simulink model "sim_model"  (R2015b)
settings: Solver=FixedStepDiscrete  SolverMode=SingleTasking  StartTime=0.0  StopTime=sim_len  FixedStep=1  RelTol=1e-3
undefined symbols (not defined in the file): A, B, C, ir_matrix, modulator_reg_1_address, modulator_reg_1_default, modulator_reg_1_num_bits, N_sub
libraries: xbsIndex_r4 x3875
(part 192 of 193)

== system sim_model/channelizer/poly_phase_filter1/filter_pipeline_89_taps3/8_taps6/one_tab_1/ring_buffer_1 ==
  reset_in : Inport
  enable_in : Inport  Port=2
  data_in : Inport  Port=3
  Register : xbsIndex_r4/Register  init=init(1)  rst=on  en=on  dbl_ovrd=off  block_type=register
  Register1 : xbsIndex_r4/Register  init=init(2)  rst=on  en=on  dbl_ovrd=off  block_type=register
  Register2 : xbsIndex_r4/Register  init=init(3)  rst=on  en=on  dbl_ovrd=off  block_type=register
  Register3 : xbsIndex_r4/Register  init=init(4)  rst=on  en=on  dbl_ovrd=off  block_type=register
  Register4 : xbsIndex_r4/Register  init=init(5)  rst=on  en=on  dbl_ovrd=off  block_type=register
  Register5 : xbsIndex_r4/Register  init=init(6)  rst=on  en=on  dbl_ovrd=off  block_type=register
  Register6 : xbsIndex_r4/Register  init=init(7)  rst=on  en=on  dbl_ovrd=off  block_type=register
  Register7 : xbsIndex_r4/Register  init=init(8)  rst=on  en=on  dbl_ovrd=off  block_type=register
  data_out : Outport
  wires:
  Register/1 -> Register1/1
  enable_in/1 -> Register7/3, Register6/3, Register5/3, Register4/3, Register3/3, Register2/3, Register1/3, Register/3
  Register7/1 -> data_out/1
  Register1/1 -> Register2/1
  Register2/1 -> Register3/1
  Register3/1 -> Register4/1
  Register5/1 -> Register6/1
  Register6/1 -> Register7/1
  Register4/1 -> Register5/1
  reset_in/1 -> Register/2, Register1/2, Register2/2, Register3/2, Register4/2, Register7/2, Register6/2, Register5/2
  data_in/1 -> Register/1

== system sim_model/channelizer/poly_phase_filter1/filter_pipeline_89_taps3/8_taps6/one_tab_1/ring_buffer_8 ==
  reset_in : Inport
  enable_in : Inport  Port=2
  data_in : Inport  Port=3
  Register : xbsIndex_r4/Register  init=init(1)  rst=on  en=on  dbl_ovrd=off  block_type=register
  Register1 : xbsIndex_r4/Register  init=init(2)  rst=on  en=on  dbl_ovrd=off  block_type=register
  Register2 : xbsIndex_r4/Register  init=init(3)  rst=on  en=on  dbl_ovrd=off  block_type=register
  Register3 : xbsIndex_r4/Register  init=init(4)  rst=on  en=on  dbl_ovrd=off  block_type=register
  Register4 : xbsIndex_r4/Register  init=init(5)  rst=on  en=on  dbl_ovrd=off  block_type=register
  Register5 : xbsIndex_r4/Register  init=init(6)  rst=on  en=on  dbl_ovrd=off  block_type=register
  Register6 : xbsIndex_r4/Register  init=init(7)  rst=on  en=on  dbl_ovrd=off  block_type=register
  Register7 : xbsIndex_r4/Register  init=init(8)  rst=on  en=on  dbl_ovrd=off  block_type=register
  data_out : Outport
  wires:
  Register/1 -> Register1/1
  enable_in/1 -> Register7/3, Register6/3, Register5/3, Register4/3, Register3/3, Register2/3, Register1/3, Register/3
  Register7/1 -> data_out/1
  Register1/1 -> Register2/1
  Register2/1 -> Register3/1
  Register3/1 -> Register4/1
  Register5/1 -> Register6/1
  Register6/1 -> Register7/1
  Register4/1 -> Register5/1
  reset_in/1 -> Register/2, Register1/2, Register2/2, Register3/2, Register4/2, Register7/2, Register6/2, Register5/2
  data_in/1 -> Register/1

== system sim_model/channelizer/poly_phase_filter1/filter_pipeline_89_taps3/8_taps6/one_tab_2/ring_buffer_1 ==
  reset_in : Inport
  enable_in : Inport  Port=2
  data_in : Inport  Port=3
  Register : xbsIndex_r4/Register  init=init(1)  rst=on  en=on  dbl_ovrd=off  block_type=register
  Register1 : xbsIndex_r4/Register  init=init(2)  rst=on  en=on  dbl_ovrd=off  block_type=register
  Register2 : xbsIndex_r4/Register  init=init(3)  rst=on  en=on  dbl_ovrd=off  block_type=register
  Register3 : xbsIndex_r4/Register  init=init(4)  rst=on  en=on  dbl_ovrd=off  block_type=register
  Register4 : xbsIndex_r4/Register  init=init(5)  rst=on  en=on  dbl_ovrd=off  block_type=register
  Register5 : xbsIndex_r4/Register  init=init(6)  rst=on  en=on  dbl_ovrd=off  block_type=register
  Register6 : xbsIndex_r4/Register  init=init(7)  rst=on  en=on  dbl_ovrd=off  block_type=register
  Register7 : xbsIndex_r4/Register  init=init(8)  rst=on  en=on  dbl_ovrd=off  block_type=register
  data_out : Outport
  wires:
  Register/1 -> Register1/1
  enable_in/1 -> Register7/3, Register6/3, Register5/3, Register4/3, Register3/3, Register2/3, Register1/3, Register/3
  Register7/1 -> data_out/1
  Register1/1 -> Register2/1
  Register2/1 -> Register3/1
  Register3/1 -> Register4/1
  Register5/1 -> Register6/1
  Register6/1 -> Register7/1
  Register4/1 -> Register5/1
  reset_in/1 -> Register/2, Register1/2, Register2/2, Register3/2, Register4/2, Register7/2, Register6/2, Register5/2
  data_in/1 -> Register/1

== system sim_model/channelizer/poly_phase_filter1/filter_pipeline_89_taps3/8_taps6/one_tab_2/ring_buffer_8 ==
  reset_in : Inport
  enable_in : Inport  Port=2
  data_in : Inport  Port=3
  Register : xbsIndex_r4/Register  init=init(1)  rst=on  en=on  dbl_ovrd=off  block_type=register
  Register1 : xbsIndex_r4/Register  init=init(2)  rst=on  en=on  dbl_ovrd=off  block_type=register
  Register2 : xbsIndex_r4/Register  init=init(3)  rst=on  en=on  dbl_ovrd=off  block_type=register
  Register3 : xbsIndex_r4/Register  init=init(4)  rst=on  en=on  dbl_ovrd=off  block_type=register
  Register4 : xbsIndex_r4/Register  init=init(5)  rst=on  en=on  dbl_ovrd=off  block_type=register
  Register5 : xbsIndex_r4/Register  init=init(6)  rst=on  en=on  dbl_ovrd=off  block_type=register
  Register6 : xbsIndex_r4/Register  init=init(7)  rst=on  en=on  dbl_ovrd=off  block_type=register
  Register7 : xbsIndex_r4/Register  init=init(8)  rst=on  en=on  dbl_ovrd=off  block_type=register
  data_out : Outport
  wires:
  Register/1 -> Register1/1
  enable_in/1 -> Register7/3, Register6/3, Register5/3, Register4/3, Register3/3, Register2/3, Register1/3, Register/3
  Register7/1 -> data_out/1
  Register1/1 -> Register2/1
  Register2/1 -> Register3/1
  Register3/1 -> Register4/1
  Register5/1 -> Register6/1
  Register6/1 -> Register7/1
  Register4/1 -> Register5/1
  reset_in/1 -> Register/2, Register1/2, Register2/2, Register3/2, Register4/2, Register7/2, Register6/2, Register5/2
  data_in/1 -> Register/1

== system sim_model/channelizer/poly_phase_filter1/filter_pipeline_89_taps3/8_taps6/one_tab_3/ring_buffer_1 ==
  reset_in : Inport
  enable_in : Inport  Port=2
  data_in : Inport  Port=3
  Register : xbsIndex_r4/Register  init=init(1)  rst=on  en=on  dbl_ovrd=off  block_type=register
  Register1 : xbsIndex_r4/Register  init=init(2)  rst=on  en=on  dbl_ovrd=off  block_type=register
  Register2 : xbsIndex_r4/Register  init=init(3)  rst=on  en=on  dbl_ovrd=off  block_type=register
  Register3 : xbsIndex_r4/Register  init=init(4)  rst=on  en=on  dbl_ovrd=off  block_type=register
  Register4 : xbsIndex_r4/Register  init=init(5)  rst=on  en=on  dbl_ovrd=off  block_type=register
  Register5 : xbsIndex_r4/Register  init=init(6)  rst=on  en=on  dbl_ovrd=off  block_type=register
  Register6 : xbsIndex_r4/Register  init=init(7)  rst=on  en=on  dbl_ovrd=off  block_type=register
  Register7 : xbsIndex_r4/Register  init=init(8)  rst=on  en=on  dbl_ovrd=off  block_type=register
  data_out : Outport
  wires:
  Register/1 -> Register1/1
  enable_in/1 -> Register7/3, Register6/3, Register5/3, Register4/3, Register3/3, Register2/3, Register1/3, Register/3
  Register7/1 -> data_out/1
  Register1/1 -> Register2/1
  Register2/1 -> Register3/1
  Register3/1 -> Register4/1
  Register5/1 -> Register6/1
  Register6/1 -> Register7/1
  Register4/1 -> Register5/1
  reset_in/1 -> Register/2, Register1/2, Register2/2, Register3/2, Register4/2, Register7/2, Register6/2, Register5/2
  data_in/1 -> Register/1

== system sim_model/channelizer/poly_phase_filter1/filter_pipeline_89_taps3/8_taps6/one_tab_3/ring_buffer_8 ==
  reset_in : Inport
  enable_in : Inport  Port=2
  data_in : Inport  Port=3
  Register : xbsIndex_r4/Register  init=init(1)  rst=on  en=on  dbl_ovrd=off  block_type=register
  Register1 : xbsIndex_r4/Register  init=init(2)  rst=on  en=on  dbl_ovrd=off  block_type=register
  Register2 : xbsIndex_r4/Register  init=init(3)  rst=on  en=on  dbl_ovrd=off  block_type=register
  Register3 : xbsIndex_r4/Register  init=init(4)  rst=on  en=on  dbl_ovrd=off  block_type=register
  Register4 : xbsIndex_r4/Register  init=init(5)  rst=on  en=on  dbl_ovrd=off  block_type=register
  Register5 : xbsIndex_r4/Register  init=init(6)  rst=on  en=on  dbl_ovrd=off  block_type=register
  Register6 : xbsIndex_r4/Register  init=init(7)  rst=on  en=on  dbl_ovrd=off  block_type=register
  Register7 : xbsIndex_r4/Register  init=init(8)  rst=on  en=on  dbl_ovrd=off  block_type=register
  data_out : Outport
  wires:
  Register/1 -> Register1/1
  enable_in/1 -> Register7/3, Register6/3, Register5/3, Register4/3, Register3/3, Register2/3, Register1/3, Register/3
  Register7/1 -> data_out/1
  Register1/1 -> Register2/1
  Register2/1 -> Register3/1
  Register3/1 -> Register4/1
  Register5/1 -> Register6/1
  Register6/1 -> Register7/1
  Register4/1 -> Register5/1
  reset_in/1 -> Register/2, Register1/2, Register2/2, Register3/2, Register4/2, Register7/2, Register6/2, Register5/2
  data_in/1 -> Register/1

== system sim_model/channelizer/poly_phase_filter1/filter_pipeline_89_taps3/8_taps6/one_tab_4/ring_buffer_1 ==
  reset_in : Inport
  enable_in : Inport  Port=2
  data_in : Inport  Port=3
  Register : xbsIndex_r4/Register  init=init(1)  rst=on  en=on  dbl_ovrd=off  block_type=register
  Register1 : xbsIndex_r4/Register  init=init(2)  rst=on  en=on  dbl_ovrd=off  block_type=register
  Register2 : xbsIndex_r4/Register  init=init(3)  rst=on  en=on  dbl_ovrd=off  block_type=register
  Register3 : xbsIndex_r4/Register  init=init(4)  rst=on  en=on  dbl_ovrd=off  block_type=register
  Register4 : xbsIndex_r4/Register  init=init(5)  rst=on  en=on  dbl_ovrd=off  block_type=register
  Register5 : xbsIndex_r4/Register  init=init(6)  rst=on  en=on  dbl_ovrd=off  block_type=register
  Register6 : xbsIndex_r4/Register  init=init(7)  rst=on  en=on  dbl_ovrd=off  block_type=register
  Register7 : xbsIndex_r4/Register  init=init(8)  rst=on  en=on  dbl_ovrd=off  block_type=register
  data_out : Outport
  wires:
  Register/1 -> Register1/1
  enable_in/1 -> Register7/3, Register6/3, Register5/3, Register4/3, Register3/3, Register2/3, Register1/3, Register/3
  Register7/1 -> data_out/1
  Register1/1 -> Register2/1
  Register2/1 -> Register3/1
  Register3/1 -> Register4/1
  Register5/1 -> Register6/1
  Register6/1 -> Register7/1
  Register4/1 -> Register5/1
  reset_in/1 -> Register/2, Register1/2, Register2/2, Register3/2, Register4/2, Register7/2, Register6/2, Register5/2
  data_in/1 -> Register/1

== system sim_model/channelizer/poly_phase_filter1/filter_pipeline_89_taps3/8_taps6/one_tab_4/ring_buffer_8 ==
  reset_in : Inport
  enable_in : Inport  Port=2
  data_in : Inport  Port=3
  Register : xbsIndex_r4/Register  init=init(1)  rst=on  en=on  dbl_ovrd=off  block_type=register
  Register1 : xbsIndex_r4/Register  init=init(2)  rst=on  en=on  dbl_ovrd=off  block_type=register
  Register2 : xbsIndex_r4/Register  init=init(3)  rst=on  en=on  dbl_ovrd=off  block_type=register
  Register3 : xbsIndex_r4/Register  init=init(4)  rst=on  en=on  dbl_ovrd=off  block_type=register
  Register4 : xbsIndex_r4/Register  init=init(5)  rst=on  en=on  dbl_ovrd=off  block_type=register
  Register5 : xbsIndex_r4/Register  init=init(6)  rst=on  en=on  dbl_ovrd=off  block_type=register
  Register6 : xbsIndex_r4/Register  init=init(7)  rst=on  en=on  dbl_ovrd=off  block_type=register
  Register7 : xbsIndex_r4/Register  init=init(8)  rst=on  en=on  dbl_ovrd=off  block_type=register
  data_out : Outport
  wires:
  Register/1 -> Register1/1
  enable_in/1 -> Register7/3, Register6/3, Register5/3, Register4/3, Register3/3, Register2/3, Register1/3, Register/3
  Register7/1 -> data_out/1
  Register1/1 -> Register2/1
  Register2/1 -> Register3/1
  Register3/1 -> Register4/1
  Register5/1 -> Register6/1
  Register6/1 -> Register7/1
  Register4/1 -> Register5/1
  reset_in/1 -> Register/2, Register1/2, Register2/2, Register3/2, Register4/2, Register7/2, Register6/2, Register5/2
  data_in/1 -> Register/1

== system sim_model/channelizer/poly_phase_filter1/filter_pipeline_89_taps3/8_taps6/one_tab_5/ring_buffer_1 ==
  reset_in : Inport
  enable_in : Inport  Port=2
  data_in : Inport  Port=3
  Register : xbsIndex_r4/Register  init=init(1)  rst=on  en=on  dbl_ovrd=off  block_type=register
  Register1 : xbsIndex_r4/Register  init=init(2)  rst=on  en=on  dbl_ovrd=off  block_type=register
  Register2 : xbsIndex_r4/Register  init=init(3)  rst=on  en=on  dbl_ovrd=off  block_type=register
  Register3 : xbsIndex_r4/Register  init=init(4)  rst=on  en=on  dbl_ovrd=off  block_type=register
  Register4 : xbsIndex_r4/Register  init=init(5)  rst=on  en=on  dbl_ovrd=off  block_type=register
  Register5 : xbsIndex_r4/Register  init=init(6)  rst=on  en=on  dbl_ovrd=off  block_type=register
  Register6 : xbsIndex_r4/Register  init=init(7)  rst=on  en=on  dbl_ovrd=off  block_type=register
  Register7 : xbsIndex_r4/Register  init=init(8)  rst=on  en=on  dbl_ovrd=off  block_type=register
  data_out : Outport
  wires:
  Register/1 -> Register1/1
  enable_in/1 -> Register7/3, Register6/3, Register5/3, Register4/3, Register3/3, Register2/3, Register1/3, Register/3
  Register7/1 -> data_out/1
  Register1/1 -> Register2/1
  Register2/1 -> Register3/1
  Register3/1 -> Register4/1
  Register5/1 -> Register6/1
  Register6/1 -> Register7/1
  Register4/1 -> Register5/1
  reset_in/1 -> Register/2, Register1/2, Register2/2, Register3/2, Register4/2, Register7/2, Register6/2, Register5/2
  data_in/1 -> Register/1

== system sim_model/channelizer/poly_phase_filter1/filter_pipeline_89_taps3/8_taps6/one_tab_5/ring_buffer_8 ==
  reset_in : Inport
  enable_in : Inport  Port=2
  data_in : Inport  Port=3
  Register : xbsIndex_r4/Register  init=init(1)  rst=on  en=on  dbl_ovrd=off  block_type=register
  Register1 : xbsIndex_r4/Register  init=init(2)  rst=on  en=on  dbl_ovrd=off  block_type=register
  Register2 : xbsIndex_r4/Register  init=init(3)  rst=on  en=on  dbl_ovrd=off  block_type=register
  Register3 : xbsIndex_r4/Register  init=init(4)  rst=on  en=on  dbl_ovrd=off  block_type=register
  Register4 : xbsIndex_r4/Register  init=init(5)  rst=on  en=on  dbl_ovrd=off  block_type=register
  Register5 : xbsIndex_r4/Register  init=init(6)  rst=on  en=on  dbl_ovrd=off  block_type=register
  Register6 : xbsIndex_r4/Register  init=init(7)  rst=on  en=on  dbl_ovrd=off  block_type=register
  Register7 : xbsIndex_r4/Register  init=init(8)  rst=on  en=on  dbl_ovrd=off  block_type=register
  data_out : Outport
  wires:
  Register/1 -> Register1/1
  enable_in/1 -> Register7/3, Register6/3, Register5/3, Register4/3, Register3/3, Register2/3, Register1/3, Register/3
  Register7/1 -> data_out/1
  Register1/1 -> Register2/1
  Register2/1 -> Register3/1
  Register3/1 -> Register4/1
  Register5/1 -> Register6/1
  Register6/1 -> Register7/1
  Register4/1 -> Register5/1
  reset_in/1 -> Register/2, Register1/2, Register2/2, Register3/2, Register4/2, Register7/2, Register6/2, Register5/2
  data_in/1 -> Register/1

== system sim_model/channelizer/poly_phase_filter1/filter_pipeline_89_taps3/8_taps6/one_tab_6/ring_buffer_1 ==
  reset_in : Inport
  enable_in : Inport  Port=2
  data_in : Inport  Port=3
  Register : xbsIndex_r4/Register  init=init(1)  rst=on  en=on  dbl_ovrd=off  block_type=register
  Register1 : xbsIndex_r4/Register  init=init(2)  rst=on  en=on  dbl_ovrd=off  block_type=register
  Register2 : xbsIndex_r4/Register  init=init(3)  rst=on  en=on  dbl_ovrd=off  block_type=register
  Register3 : xbsIndex_r4/Register  init=init(4)  rst=on  en=on  dbl_ovrd=off  block_type=register
  Register4 : xbsIndex_r4/Register  init=init(5)  rst=on  en=on  dbl_ovrd=off  block_type=register
  Register5 : xbsIndex_r4/Register  init=init(6)  rst=on  en=on  dbl_ovrd=off  block_type=register
  Register6 : xbsIndex_r4/Register  init=init(7)  rst=on  en=on  dbl_ovrd=off  block_type=register
  Register7 : xbsIndex_r4/Register  init=init(8)  rst=on  en=on  dbl_ovrd=off  block_type=register
  data_out : Outport
  wires:
  Register/1 -> Register1/1
  enable_in/1 -> Register7/3, Register6/3, Register5/3, Register4/3, Register3/3, Register2/3, Register1/3, Register/3
  Register7/1 -> data_out/1
  Register1/1 -> Register2/1
  Register2/1 -> Register3/1
  Register3/1 -> Register4/1
  Register5/1 -> Register6/1
  Register6/1 -> Register7/1
  Register4/1 -> Register5/1
  reset_in/1 -> Register/2, Register1/2, Register2/2, Register3/2, Register4/2, Register7/2, Register6/2, Register5/2
  data_in/1 -> Register/1

== system sim_model/channelizer/poly_phase_filter1/filter_pipeline_89_taps3/8_taps6/one_tab_6/ring_buffer_8 ==
  reset_in : Inport
  enable_in : Inport  Port=2
  data_in : Inport  Port=3
  Register : xbsIndex_r4/Register  init=init(1)  rst=on  en=on  dbl_ovrd=off  block_type=register
  Register1 : xbsIndex_r4/Register  init=init(2)  rst=on  en=on  dbl_ovrd=off  block_type=register
  Register2 : xbsIndex_r4/Register  init=init(3)  rst=on  en=on  dbl_ovrd=off  block_type=register
  Register3 : xbsIndex_r4/Register  init=init(4)  rst=on  en=on  dbl_ovrd=off  block_type=register
  Register4 : xbsIndex_r4/Register  init=init(5)  rst=on  en=on  dbl_ovrd=off  block_type=register
  Register5 : xbsIndex_r4/Register  init=init(6)  rst=on  en=on  dbl_ovrd=off  block_type=register
  Register6 : xbsIndex_r4/Register  init=init(7)  rst=on  en=on  dbl_ovrd=off  block_type=register
  Register7 : xbsIndex_r4/Register  init=init(8)  rst=on  en=on  dbl_ovrd=off  block_type=register
  data_out : Outport
  wires:
  Register/1 -> Register1/1
  enable_in/1 -> Register7/3, Register6/3, Register5/3, Register4/3, Register3/3, Register2/3, Register1/3, Register/3
  Register7/1 -> data_out/1
  Register1/1 -> Register2/1
  Register2/1 -> Register3/1
  Register3/1 -> Register4/1
  Register5/1 -> Register6/1
  Register6/1 -> Register7/1
  Register4/1 -> Register5/1
  reset_in/1 -> Register/2, Register1/2, Register2/2, Register3/2, Register4/2, Register7/2, Register6/2, Register5/2
  data_in/1 -> Register/1

== system sim_model/channelizer/poly_phase_filter1/filter_pipeline_89_taps3/8_taps6/one_tab_7/ring_buffer_1 ==
  reset_in : Inport
  enable_in : Inport  Port=2
  data_in : Inport  Port=3
  Register : xbsIndex_r4/Register  init=init(1)  rst=on  en=on  dbl_ovrd=off  block_type=register
  Register1 : xbsIndex_r4/Register  init=init(2)  rst=on  en=on  dbl_ovrd=off  block_type=register
  Register2 : xbsIndex_r4/Register  init=init(3)  rst=on  en=on  dbl_ovrd=off  block_type=register
  Register3 : xbsIndex_r4/Register  init=init(4)  rst=on  en=on  dbl_ovrd=off  block_type=register
  Register4 : xbsIndex_r4/Register  init=init(5)  rst=on  en=on  dbl_ovrd=off  block_type=register
  Register5 : xbsIndex_r4/Register  init=init(6)  rst=on  en=on  dbl_ovrd=off  block_type=register
  Register6 : xbsIndex_r4/Register  init=init(7)  rst=on  en=on  dbl_ovrd=off  block_type=register
  Register7 : xbsIndex_r4/Register  init=init(8)  rst=on  en=on  dbl_ovrd=off  block_type=register
  data_out : Outport
  wires:
  Register/1 -> Register1/1
  enable_in/1 -> Register7/3, Register6/3, Register5/3, Register4/3, Register3/3, Register2/3, Register1/3, Register/3
  Register7/1 -> data_out/1
  Register1/1 -> Register2/1
  Register2/1 -> Register3/1
  Register3/1 -> Register4/1
  Register5/1 -> Register6/1
  Register6/1 -> Register7/1
  Register4/1 -> Register5/1
  reset_in/1 -> Register/2, Register1/2, Register2/2, Register3/2, Register4/2, Register7/2, Register6/2, Register5/2
  data_in/1 -> Register/1

== system sim_model/channelizer/poly_phase_filter1/filter_pipeline_89_taps3/8_taps6/one_tab_7/ring_buffer_8 ==
  reset_in : Inport
  enable_in : Inport  Port=2
  data_in : Inport  Port=3
  Register : xbsIndex_r4/Register  init=init(1)  rst=on  en=on  dbl_ovrd=off  block_type=register
  Register1 : xbsIndex_r4/Register  init=init(2)  rst=on  en=on  dbl_ovrd=off  block_type=register
  Register2 : xbsIndex_r4/Register  init=init(3)  rst=on  en=on  dbl_ovrd=off  block_type=register
  Register3 : xbsIndex_r4/Register  init=init(4)  rst=on  en=on  dbl_ovrd=off  block_type=register
  Register4 : xbsIndex_r4/Register  init=init(5)  rst=on  en=on  dbl_ovrd=off  block_type=register
  Register5 : xbsIndex_r4/Register  init=init(6)  rst=on  en=on  dbl_ovrd=off  block_type=register
  Register6 : xbsIndex_r4/Register  init=init(7)  rst=on  en=on  dbl_ovrd=off  block_type=register
  Register7 : xbsIndex_r4/Register  init=init(8)  rst=on  en=on  dbl_ovrd=off  block_type=register
  data_out : Outport
  wires:
  Register/1 -> Register1/1
  enable_in/1 -> Register7/3, Register6/3, Register5/3, Register4/3, Register3/3, Register2/3, Register1/3, Register/3
  Register7/1 -> data_out/1
  Register1/1 -> Register2/1
  Register2/1 -> Register3/1
  Register3/1 -> Register4/1
  Register5/1 -> Register6/1
  Register6/1 -> Register7/1
  Register4/1 -> Register5/1
  reset_in/1 -> Register/2, Register1/2, Register2/2, Register3/2, Register4/2, Register7/2, Register6/2, Register5/2
  data_in/1 -> Register/1

== system sim_model/channelizer/poly_phase_filter1/filter_pipeline_89_taps3/8_taps6/one_tab_8/ring_buffer_1 ==
  reset_in : Inport
  enable_in : Inport  Port=2
  data_in : Inport  Port=3
  Register : xbsIndex_r4/Register  init=init(1)  rst=on  en=on  dbl_ovrd=off  block_type=register
  Register1 : xbsIndex_r4/Register  init=init(2)  rst=on  en=on  dbl_ovrd=off  block_type=register
  Register2 : xbsIndex_r4/Register  init=init(3)  rst=on  en=on  dbl_ovrd=off  block_type=register
  Register3 : xbsIndex_r4/Register  init=init(4)  rst=on  en=on  dbl_ovrd=off  block_type=register
  Register4 : xbsIndex_r4/Register  init=init(5)  rst=on  en=on  dbl_ovrd=off  block_type=register
  Register5 : xbsIndex_r4/Register  init=init(6)  rst=on  en=on  dbl_ovrd=off  block_type=register
  Register6 : xbsIndex_r4/Register  init=init(7)  rst=on  en=on  dbl_ovrd=off  block_type=register
  Register7 : xbsIndex_r4/Register  init=init(8)  rst=on  en=on  dbl_ovrd=off  block_type=register
  data_out : Outport
  wires:
  Register/1 -> Register1/1
  enable_in/1 -> Register7/3, Register6/3, Register5/3, Register4/3, Register3/3, Register2/3, Register1/3, Register/3
  Register7/1 -> data_out/1
  Register1/1 -> Register2/1
  Register2/1 -> Register3/1
  Register3/1 -> Register4/1
  Register5/1 -> Register6/1
  Register6/1 -> Register7/1
  Register4/1 -> Register5/1
  reset_in/1 -> Register/2, Register1/2, Register2/2, Register3/2, Register4/2, Register7/2, Register6/2, Register5/2
  data_in/1 -> Register/1

== system sim_model/channelizer/poly_phase_filter1/filter_pipeline_89_taps3/8_taps6/one_tab_8/ring_buffer_8 ==
  reset_in : Inport
  enable_in : Inport  Port=2
  data_in : Inport  Port=3
  Register : xbsIndex_r4/Register  init=init(1)  rst=on  en=on  dbl_ovrd=off  block_type=register
  Register1 : xbsIndex_r4/Register  init=init(2)  rst=on  en=on  dbl_ovrd=off  block_type=register
  Register2 : xbsIndex_r4/Register  init=init(3)  rst=on  en=on  dbl_ovrd=off  block_type=register
  Register3 : xbsIndex_r4/Register  init=init(4)  rst=on  en=on  dbl_ovrd=off  block_type=register
  Register4 : xbsIndex_r4/Register  init=init(5)  rst=on  en=on  dbl_ovrd=off  block_type=register
  Register5 : xbsIndex_r4/Register  init=init(6)  rst=on  en=on  dbl_ovrd=off  block_type=register
  Register6 : xbsIndex_r4/Register  init=init(7)  rst=on  en=on  dbl_ovrd=off  block_type=register
  Register7 : xbsIndex_r4/Register  init=init(8)  rst=on  en=on  dbl_ovrd=off  block_type=register
  data_out : Outport
  wires:
  Register/1 -> Register1/1
  enable_in/1 -> Register7/3, Register6/3, Register5/3, Register4/3, Register3/3, Register2/3, Register1/3, Register/3
  Register7/1 -> data_out/1
  Register1/1 -> Register2/1
  Register2/1 -> Register3/1
  Register3/1 -> Register4/1
  Register5/1 -> Register6/1
  Register6/1 -> Register7/1
  Register4/1 -> Register5/1
  reset_in/1 -> Register/2, Register1/2, Register2/2, Register3/2, Register4/2, Register7/2, Register6/2, Register5/2
  data_in/1 -> Register/1

== system sim_model/channelizer/poly_phase_filter1/filter_pipeline_89_taps3/8_taps7/one_tab_1/ring_buffer_1 ==
  reset_in : Inport
  enable_in : Inport  Port=2
  data_in : Inport  Port=3
  Register : xbsIndex_r4/Register  init=init(1)  rst=on  en=on  dbl_ovrd=off  block_type=register
  Register1 : xbsIndex_r4/Register  init=init(2)  rst=on  en=on  dbl_ovrd=off  block_type=register
  Register2 : xbsIndex_r4/Register  init=init(3)  rst=on  en=on  dbl_ovrd=off  block_type=register
  Register3 : xbsIndex_r4/Register  init=init(4)  rst=on  en=on  dbl_ovrd=off  block_type=register
  Register4 : xbsIndex_r4/Register  init=init(5)  rst=on  en=on  dbl_ovrd=off  block_type=register
  Register5 : xbsIndex_r4/Register  init=init(6)  rst=on  en=on  dbl_ovrd=off  block_type=register
  Register6 : xbsIndex_r4/Register  init=init(7)  rst=on  en=on  dbl_ovrd=off  block_type=register
  Register7 : xbsIndex_r4/Register  init=init(8)  rst=on  en=on  dbl_ovrd=off  block_type=register
  data_out : Outport
  wires:
  Register/1 -> Register1/1
  enable_in/1 -> Register7/3, Register6/3, Register5/3, Register4/3, Register3/3, Register2/3, Register1/3, Register/3
  Register7/1 -> data_out/1
  Register1/1 -> Register2/1
  Register2/1 -> Register3/1
  Register3/1 -> Register4/1
  Register5/1 -> Register6/1
  Register6/1 -> Register7/1
  Register4/1 -> Register5/1
  reset_in/1 -> Register/2, Register1/2, Register2/2, Register3/2, Register4/2, Register7/2, Register6/2, Register5/2
  data_in/1 -> Register/1

== system sim_model/channelizer/poly_phase_filter1/filter_pipeline_89_taps3/8_taps7/one_tab_1/ring_buffer_8 ==
  reset_in : Inport
  enable_in : Inport  Port=2
  data_in : Inport  Port=3
  Register : xbsIndex_r4/Register  init=init(1)  rst=on  en=on  dbl_ovrd=off  block_type=register
  Register1 : xbsIndex_r4/Register  init=init(2)  rst=on  en=on  dbl_ovrd=off  block_type=register
  Register2 : xbsIndex_r4/Register  init=init(3)  rst=on  en=on  dbl_ovrd=off  block_type=register
  Register3 : xbsIndex_r4/Register  init=init(4)  rst=on  en=on  dbl_ovrd=off  block_type=register
  Register4 : xbsIndex_r4/Register  init=init(5)  rst=on  en=on  dbl_ovrd=off  block_type=register
  Register5 : xbsIndex_r4/Register  init=init(6)  rst=on  en=on  dbl_ovrd=off  block_type=register
  Register6 : xbsIndex_r4/Register  init=init(7)  rst=on  en=on  dbl_ovrd=off  block_type=register
  Register7 : xbsIndex_r4/Register  init=init(8)  rst=on  en=on  dbl_ovrd=off  block_type=register
  data_out : Outport
  wires:
  Register/1 -> Register1/1
  enable_in/1 -> Register7/3, Register6/3, Register5/3, Register4/3, Register3/3, Register2/3, Register1/3, Register/3
  Register7/1 -> data_out/1
  Register1/1 -> Register2/1
  Register2/1 -> Register3/1
  Register3/1 -> Register4/1
  Register5/1 -> Register6/1
  Register6/1 -> Register7/1
  Register4/1 -> Register5/1
  reset_in/1 -> Register/2, Register1/2, Register2/2, Register3/2, Register4/2, Register7/2, Register6/2, Register5/2
  data_in/1 -> Register/1

== system sim_model/channelizer/poly_phase_filter1/filter_pipeline_89_taps3/8_taps7/one_tab_2/ring_buffer_1 ==
  reset_in : Inport
  enable_in : Inport  Port=2
  data_in : Inport  Port=3
  Register : xbsIndex_r4/Register  init=init(1)  rst=on  en=on  dbl_ovrd=off  block_type=register
  Register1 : xbsIndex_r4/Register  init=init(2)  rst=on  en=on  dbl_ovrd=off  block_type=register
  Register2 : xbsIndex_r4/Register  init=init(3)  rst=on  en=on  dbl_ovrd=off  block_type=register
  Register3 : xbsIndex_r4/Register  init=init(4)  rst=on  en=on  dbl_ovrd=off  block_type=register
  Register4 : xbsIndex_r4/Register  init=init(5)  rst=on  en=on  dbl_ovrd=off  block_type=register
  Register5 : xbsIndex_r4/Register  init=init(6)  rst=on  en=on  dbl_ovrd=off  block_type=register
  Register6 : xbsIndex_r4/Register  init=init(7)  rst=on  en=on  dbl_ovrd=off  block_type=register
  Register7 : xbsIndex_r4/Register  init=init(8)  rst=on  en=on  dbl_ovrd=off  block_type=register
  data_out : Outport
  wires:
  Register/1 -> Register1/1
  enable_in/1 -> Register7/3, Register6/3, Register5/3, Register4/3, Register3/3, Register2/3, Register1/3, Register/3
  Register7/1 -> data_out/1
  Register1/1 -> Register2/1
  Register2/1 -> Register3/1
  Register3/1 -> Register4/1
  Register5/1 -> Register6/1
  Register6/1 -> Register7/1
  Register4/1 -> Register5/1
  reset_in/1 -> Register/2, Register1/2, Register2/2, Register3/2, Register4/2, Register7/2, Register6/2, Register5/2
  data_in/1 -> Register/1

== system sim_model/channelizer/poly_phase_filter1/filter_pipeline_89_taps3/8_taps7/one_tab_2/ring_buffer_8 ==
  reset_in : Inport
  enable_in : Inport  Port=2
  data_in : Inport  Port=3
  Register : xbsIndex_r4/Register  init=init(1)  rst=on  en=on  dbl_ovrd=off  block_type=register
  Register1 : xbsIndex_r4/Register  init=init(2)  rst=on  en=on  dbl_ovrd=off  block_type=register
  Register2 : xbsIndex_r4/Register  init=init(3)  rst=on  en=on  dbl_ovrd=off  block_type=register
  Register3 : xbsIndex_r4/Register  init=init(4)  rst=on  en=on  dbl_ovrd=off  block_type=register
  Register4 : xbsIndex_r4/Register  init=init(5)  rst=on  en=on  dbl_ovrd=off  block_type=register
  Register5 : xbsIndex_r4/Register  init=init(6)  rst=on  en=on  dbl_ovrd=off  block_type=register
  Register6 : xbsIndex_r4/Register  init=init(7)  rst=on  en=on  dbl_ovrd=off  block_type=register
  Register7 : xbsIndex_r4/Register  init=init(8)  rst=on  en=on  dbl_ovrd=off  block_type=register
  data_out : Outport
  wires:
  Register/1 -> Register1/1
  enable_in/1 -> Register7/3, Register6/3, Register5/3, Register4/3, Register3/3, Register2/3, Register1/3, Register/3
  Register7/1 -> data_out/1
  Register1/1 -> Register2/1
  Register2/1 -> Register3/1
  Register3/1 -> Register4/1
  Register5/1 -> Register6/1
  Register6/1 -> Register7/1
  Register4/1 -> Register5/1
  reset_in/1 -> Register/2, Register1/2, Register2/2, Register3/2, Register4/2, Register7/2, Register6/2, Register5/2
  data_in/1 -> Register/1

== system sim_model/channelizer/poly_phase_filter1/filter_pipeline_89_taps3/8_taps7/one_tab_3/ring_buffer_1 ==
  reset_in : Inport
  enable_in : Inport  Port=2
  data_in : Inport  Port=3
  Register : xbsIndex_r4/Register  init=init(1)  rst=on  en=on  dbl_ovrd=off  block_type=register
  Register1 : xbsIndex_r4/Register  init=init(2)  rst=on  en=on  dbl_ovrd=off  block_type=register
  Register2 : xbsIndex_r4/Register  init=init(3)  rst=on  en=on  dbl_ovrd=off  block_type=register
  Register3 : xbsIndex_r4/Register  init=init(4)  rst=on  en=on  dbl_ovrd=off  block_type=register
  Register4 : xbsIndex_r4/Register  init=init(5)  rst=on  en=on  dbl_ovrd=off  block_type=register
  Register5 : xbsIndex_r4/Register  init=init(6)  rst=on  en=on  dbl_ovrd=off  block_type=register
  Register6 : xbsIndex_r4/Register  init=init(7)  rst=on  en=on  dbl_ovrd=off  block_type=register
  Register7 : xbsIndex_r4/Register  init=init(8)  rst=on  en=on  dbl_ovrd=off  block_type=register
  data_out : Outport
  wires:
  Register/1 -> Register1/1
  enable_in/1 -> Register7/3, Register6/3, Register5/3, Register4/3, Register3/3, Register2/3, Register1/3, Register/3
  Register7/1 -> data_out/1
  Register1/1 -> Register2/1
  Register2/1 -> Register3/1
  Register3/1 -> Register4/1
  Register5/1 -> Register6/1
  Register6/1 -> Register7/1
  Register4/1 -> Register5/1
  reset_in/1 -> Register/2, Register1/2, Register2/2, Register3/2, Register4/2, Register7/2, Register6/2, Register5/2
  data_in/1 -> Register/1

== system sim_model/channelizer/poly_phase_filter1/filter_pipeline_89_taps3/8_taps7/one_tab_3/ring_buffer_8 ==
  reset_in : Inport
  enable_in : Inport  Port=2
  data_in : Inport  Port=3
  Register : xbsIndex_r4/Register  init=init(1)  rst=on  en=on  dbl_ovrd=off  block_type=register
  Register1 : xbsIndex_r4/Register  init=init(2)  rst=on  en=on  dbl_ovrd=off  block_type=register
  Register2 : xbsIndex_r4/Register  init=init(3)  rst=on  en=on  dbl_ovrd=off  block_type=register
  Register3 : xbsIndex_r4/Register  init=init(4)  rst=on  en=on  dbl_ovrd=off  block_type=register
  Register4 : xbsIndex_r4/Register  init=init(5)  rst=on  en=on  dbl_ovrd=off  block_type=register
  Register5 : xbsIndex_r4/Register  init=init(6)  rst=on  en=on  dbl_ovrd=off  block_type=register
  Register6 : xbsIndex_r4/Register  init=init(7)  rst=on  en=on  dbl_ovrd=off  block_type=register
  Register7 : xbsIndex_r4/Register  init=init(8)  rst=on  en=on  dbl_ovrd=off  block_type=register
  data_out : Outport
  wires:
  Register/1 -> Register1/1
  enable_in/1 -> Register7/3, Register6/3, Register5/3, Register4/3, Register3/3, Register2/3, Register1/3, Register/3
  Register7/1 -> data_out/1
  Register1/1 -> Register2/1
  Register2/1 -> Register3/1
  Register3/1 -> Register4/1
  Register5/1 -> Register6/1
  Register6/1 -> Register7/1
  Register4/1 -> Register5/1
  reset_in/1 -> Register/2, Register1/2, Register2/2, Register3/2, Register4/2, Register7/2, Register6/2, Register5/2
  data_in/1 -> Register/1

== system sim_model/channelizer/poly_phase_filter1/filter_pipeline_89_taps3/8_taps7/one_tab_4/ring_buffer_1 ==
  reset_in : Inport
  enable_in : Inport  Port=2
  data_in : Inport  Port=3
  Register : xbsIndex_r4/Register  init=init(1)  rst=on  en=on  dbl_ovrd=off  block_type=register
  Register1 : xbsIndex_r4/Register  init=init(2)  rst=on  en=on  dbl_ovrd=off  block_type=register
  Register2 : xbsIndex_r4/Register  init=init(3)  rst=on  en=on  dbl_ovrd=off  block_type=register
  Register3 : xbsIndex_r4/Register  init=init(4)  rst=on  en=on  dbl_ovrd=off  block_type=register
  Register4 : xbsIndex_r4/Register  init=init(5)  rst=on  en=on  dbl_ovrd=off  block_type=register
  Register5 : xbsIndex_r4/Register  init=init(6)  rst=on  en=on  dbl_ovrd=off  block_type=register
  Register6 : xbsIndex_r4/Register  init=init(7)  rst=on  en=on  dbl_ovrd=off  block_type=register
  Register7 : xbsIndex_r4/Register  init=init(8)  rst=on  en=on  dbl_ovrd=off  block_type=register
  data_out : Outport
  wires:
  Register/1 -> Register1/1
  enable_in/1 -> Register7/3, Register6/3, Register5/3, Register4/3, Register3/3, Register2/3, Register1/3, Register/3
  Register7/1 -> data_out/1
  Register1/1 -> Register2/1
  Register2/1 -> Register3/1
  Register3/1 -> Register4/1
  Register5/1 -> Register6/1
  Register6/1 -> Register7/1
  Register4/1 -> Register5/1
  reset_in/1 -> Register/2, Register1/2, Register2/2, Register3/2, Register4/2, Register7/2, Register6/2, Register5/2
  data_in/1 -> Register/1

== system sim_model/channelizer/poly_phase_filter1/filter_pipeline_89_taps3/8_taps7/one_tab_4/ring_buffer_8 ==
  reset_in : Inport
  enable_in : Inport  Port=2
  data_in : Inport  Port=3
  Register : xbsIndex_r4/Register  init=init(1)  rst=on  en=on  dbl_ovrd=off  block_type=register
  Register1 : xbsIndex_r4/Register  init=init(2)  rst=on  en=on  dbl_ovrd=off  block_type=register
  Register2 : xbsIndex_r4/Register  init=init(3)  rst=on  en=on  dbl_ovrd=off  block_type=register
  Register3 : xbsIndex_r4/Register  init=init(4)  rst=on  en=on  dbl_ovrd=off  block_type=register
  Register4 : xbsIndex_r4/Register  init=init(5)  rst=on  en=on  dbl_ovrd=off  block_type=register
  Register5 : xbsIndex_r4/Register  init=init(6)  rst=on  en=on  dbl_ovrd=off  block_type=register
  Register6 : xbsIndex_r4/Register  init=init(7)  rst=on  en=on  dbl_ovrd=off  block_type=register
  Register7 : xbsIndex_r4/Register  init=init(8)  rst=on  en=on  dbl_ovrd=off  block_type=register
  data_out : Outport
  wires:
  Register/1 -> Register1/1
  enable_in/1 -> Register7/3, Register6/3, Register5/3, Register4/3, Register3/3, Register2/3, Register1/3, Register/3
  Register7/1 -> data_out/1
  Register1/1 -> Register2/1
  Register2/1 -> Register3/1
  Register3/1 -> Register4/1
  Register5/1 -> Register6/1
  Register6/1 -> Register7/1
  Register4/1 -> Register5/1
  reset_in/1 -> Register/2, Register1/2, Register2/2, Register3/2, Register4/2, Register7/2, Register6/2, Register5/2
  data_in/1 -> Register/1

== system sim_model/channelizer/poly_phase_filter1/filter_pipeline_89_taps3/8_taps7/one_tab_5/ring_buffer_1 ==
  reset_in : Inport
  enable_in : Inport  Port=2
  data_in : Inport  Port=3
  Register : xbsIndex_r4/Register  init=init(1)  rst=on  en=on  dbl_ovrd=off  block_type=register
  Register1 : xbsIndex_r4/Register  init=init(2)  rst=on  en=on  dbl_ovrd=off  block_type=register
  Register2 : xbsIndex_r4/Register  init=init(3)  rst=on  en=on  dbl_ovrd=off  block_type=register
  Register3 : xbsIndex_r4/Register  init=init(4)  rst=on  en=on  dbl_ovrd=off  block_type=register
  Register4 : xbsIndex_r4/Register  init=init(5)  rst=on  en=on  dbl_ovrd=off  block_type=register
  Register5 : xbsIndex_r4/Register  init=init(6)  rst=on  en=on  dbl_ovrd=off  block_type=register
  Register6 : xbsIndex_r4/Register  init=init(7)  rst=on  en=on  dbl_ovrd=off  block_type=register
  Register7 : xbsIndex_r4/Register  init=init(8)  rst=on  en=on  dbl_ovrd=off  block_type=register
  data_out : Outport
  wires:
  Register/1 -> Register1/1
  enable_in/1 -> Register7/3, Register6/3, Register5/3, Register4/3, Register3/3, Register2/3, Register1/3, Register/3
  Register7/1 -> data_out/1
  Register1/1 -> Register2/1
  Register2/1 -> Register3/1
  Register3/1 -> Register4/1
  Register5/1 -> Register6/1
  Register6/1 -> Register7/1
  Register4/1 -> Register5/1
  reset_in/1 -> Register/2, Register1/2, Register2/2, Register3/2, Register4/2, Register7/2, Register6/2, Register5/2
  data_in/1 -> Register/1

== system sim_model/channelizer/poly_phase_filter1/filter_pipeline_89_taps3/8_taps7/one_tab_5/ring_buffer_8 ==
  reset_in : Inport
  enable_in : Inport  Port=2
  data_in : Inport  Port=3
  Register : xbsIndex_r4/Register  init=init(1)  rst=on  en=on  dbl_ovrd=off  block_type=register
  Register1 : xbsIndex_r4/Register  init=init(2)  rst=on  en=on  dbl_ovrd=off  block_type=register
  Register2 : xbsIndex_r4/Register  init=init(3)  rst=on  en=on  dbl_ovrd=off  block_type=register
  Register3 : xbsIndex_r4/Register  init=init(4)  rst=on  en=on  dbl_ovrd=off  block_type=register
  Register4 : xbsIndex_r4/Register  init=init(5)  rst=on  en=on  dbl_ovrd=off  block_type=register
  Register5 : xbsIndex_r4/Register  init=init(6)  rst=on  en=on  dbl_ovrd=off  block_type=register
  Register6 : xbsIndex_r4/Register  init=init(7)  rst=on  en=on  dbl_ovrd=off  block_type=register
  Register7 : xbsIndex_r4/Register  init=init(8)  rst=on  en=on  dbl_ovrd=off  block_type=register
  data_out : Outport
  wires:
  Register/1 -> Register1/1
  enable_in/1 -> Register7/3, Register6/3, Register5/3, Register4/3, Register3/3, Register2/3, Register1/3, Register/3
  Register7/1 -> data_out/1
  Register1/1 -> Register2/1
  Register2/1 -> Register3/1
  Register3/1 -> Register4/1
  Register5/1 -> Register6/1
  Register6/1 -> Register7/1
  Register4/1 -> Register5/1
  reset_in/1 -> Register/2, Register1/2, Register2/2, Register3/2, Register4/2, Register7/2, Register6/2, Register5/2
  data_in/1 -> Register/1

== system sim_model/channelizer/poly_phase_filter1/filter_pipeline_89_taps3/8_taps7/one_tab_6/ring_buffer_1 ==
  reset_in : Inport
  enable_in : Inport  Port=2
  data_in : Inport  Port=3
  Register : xbsIndex_r4/Register  init=init(1)  rst=on  en=on  dbl_ovrd=off  block_type=register
  Register1 : xbsIndex_r4/Register  init=init(2)  rst=on  en=on  dbl_ovrd=off  block_type=register
  Register2 : xbsIndex_r4/Register  init=init(3)  rst=on  en=on  dbl_ovrd=off  block_type=register
  Register3 : xbsIndex_r4/Register  init=init(4)  rst=on  en=on  dbl_ovrd=off  block_type=register
  Register4 : xbsIndex_r4/Register  init=init(5)  rst=on  en=on  dbl_ovrd=off  block_type=register
  Register5 : xbsIndex_r4/Register  init=init(6)  rst=on  en=on  dbl_ovrd=off  block_type=register
  Register6 : xbsIndex_r4/Register  init=init(7)  rst=on  en=on  dbl_ovrd=off  block_type=register
  Register7 : xbsIndex_r4/Register  init=init(8)  rst=on  en=on  dbl_ovrd=off  block_type=register
  data_out : Outport
  wires:
  Register/1 -> Register1/1
  enable_in/1 -> Register7/3, Register6/3, Register5/3, Register4/3, Register3/3, Register2/3, Register1/3, Register/3
  Register7/1 -> data_out/1
  Register1/1 -> Register2/1
  Register2/1 -> Register3/1
  Register3/1 -> Register4/1
  Register5/1 -> Register6/1
  Register6/1 -> Register7/1
  Register4/1 -> Register5/1
  reset_in/1 -> Register/2, Register1/2, Register2/2, Register3/2, Register4/2, Register7/2, Register6/2, Register5/2
  data_in/1 -> Register/1

== system sim_model/channelizer/poly_phase_filter1/filter_pipeline_89_taps3/8_taps7/one_tab_6/ring_buffer_8 ==
  reset_in : Inport
  enable_in : Inport  Port=2
  data_in : Inport  Port=3
  Register : xbsIndex_r4/Register  init=init(1)  rst=on  en=on  dbl_ovrd=off  block_type=register
  Register1 : xbsIndex_r4/Register  init=init(2)  rst=on  en=on  dbl_ovrd=off  block_type=register
  Register2 : xbsIndex_r4/Register  init=init(3)  rst=on  en=on  dbl_ovrd=off  block_type=register
  Register3 : xbsIndex_r4/Register  init=init(4)  rst=on  en=on  dbl_ovrd=off  block_type=register
  Register4 : xbsIndex_r4/Register  init=init(5)  rst=on  en=on  dbl_ovrd=off  block_type=register
  Register5 : xbsIndex_r4/Register  init=init(6)  rst=on  en=on  dbl_ovrd=off  block_type=register
  Register6 : xbsIndex_r4/Register  init=init(7)  rst=on  en=on  dbl_ovrd=off  block_type=register
  Register7 : xbsIndex_r4/Register  init=init(8)  rst=on  en=on  dbl_ovrd=off  block_type=register
  data_out : Outport
  wires:
  Register/1 -> Register1/1
  enable_in/1 -> Register7/3, Register6/3, Register5/3, Register4/3, Register3/3, Register2/3, Register1/3, Register/3
  Register7/1 -> data_out/1
  Register1/1 -> Register2/1
  Register2/1 -> Register3/1
  Register3/1 -> Register4/1
  Register5/1 -> Register6/1
  Register6/1 -> Register7/1
  Register4/1 -> Register5/1
  reset_in/1 -> Register/2, Register1/2, Register2/2, Register3/2, Register4/2, Register7/2, Register6/2, Register5/2
  data_in/1 -> Register/1

== system sim_model/channelizer/poly_phase_filter1/filter_pipeline_89_taps3/8_taps7/one_tab_7/ring_buffer_1 ==
  reset_in : Inport
  enable_in : Inport  Port=2
  data_in : Inport  Port=3
  Register : xbsIndex_r4/Register  init=init(1)  rst=on  en=on  dbl_ovrd=off  block_type=register
  Register1 : xbsIndex_r4/Register  init=init(2)  rst=on  en=on  dbl_ovrd=off  block_type=register
  Register2 : xbsIndex_r4/Register  init=init(3)  rst=on  en=on  dbl_ovrd=off  block_type=register
  Register3 : xbsIndex_r4/Register  init=init(4)  rst=on  en=on  dbl_ovrd=off  block_type=register
  Register4 : xbsIndex_r4/Register  init=init(5)  rst=on  en=on  dbl_ovrd=off  block_type=register
  Register5 : xbsIndex_r4/Register  init=init(6)  rst=on  en=on  dbl_ovrd=off  block_type=register
  Register6 : xbsIndex_r4/Register  init=init(7)  rst=on  en=on  dbl_ovrd=off  block_type=register
  Register7 : xbsIndex_r4/Register  init=init(8)  rst=on  en=on  dbl_ovrd=off  block_type=register
  data_out : Outport
  wires:
  Register/1 -> Register1/1
  enable_in/1 -> Register7/3, Register6/3, Register5/3, Register4/3, Register3/3, Register2/3, Register1/3, Register/3
  Register7/1 -> data_out/1
  Register1/1 -> Register2/1
  Register2/1 -> Register3/1
  Register3/1 -> Register4/1
  Register5/1 -> Register6/1
  Register6/1 -> Register7/1
  Register4/1 -> Register5/1
  reset_in/1 -> Register/2, Register1/2, Register2/2, Register3/2, Register4/2, Register7/2, Register6/2, Register5/2
  data_in/1 -> Register/1

== system sim_model/channelizer/poly_phase_filter1/filter_pipeline_89_taps3/8_taps7/one_tab_7/ring_buffer_8 ==
  reset_in : Inport
  enable_in : Inport  Port=2
  data_in : Inport  Port=3
  Register : xbsIndex_r4/Register  init=init(1)  rst=on  en=on  dbl_ovrd=off  block_type=register
  Register1 : xbsIndex_r4/Register  init=init(2)  rst=on  en=on  dbl_ovrd=off  block_type=register
  Register2 : xbsIndex_r4/Register  init=init(3)  rst=on  en=on  dbl_ovrd=off  block_type=register
  Register3 : xbsIndex_r4/Register  init=init(4)  rst=on  en=on  dbl_ovrd=off  block_type=register
  Register4 : xbsIndex_r4/Register  init=init(5)  rst=on  en=on  dbl_ovrd=off  block_type=register
  Register5 : xbsIndex_r4/Register  init=init(6)  rst=on  en=on  dbl_ovrd=off  block_type=register
  Register6 : xbsIndex_r4/Register  init=init(7)  rst=on  en=on  dbl_ovrd=off  block_type=register
  Register7 : xbsIndex_r4/Register  init=init(8)  rst=on  en=on  dbl_ovrd=off  block_type=register
  data_out : Outport
  wires:
  Register/1 -> Register1/1
  enable_in/1 -> Register7/3, Register6/3, Register5/3, Register4/3, Register3/3, Register2/3, Register1/3, Register/3
  Register7/1 -> data_out/1
  Register1/1 -> Register2/1
  Register2/1 -> Register3/1
  Register3/1 -> Register4/1
  Register5/1 -> Register6/1
  Register6/1 -> Register7/1
  Register4/1 -> Register5/1
  reset_in/1 -> Register/2, Register1/2, Register2/2, Register3/2, Register4/2, Register7/2, Register6/2, Register5/2
  data_in/1 -> Register/1

== system sim_model/channelizer/poly_phase_filter1/filter_pipeline_89_taps3/8_taps7/one_tab_8/ring_buffer_1 ==
  reset_in : Inport
  enable_in : Inport  Port=2
  data_in : Inport  Port=3
  Register : xbsIndex_r4/Register  init=init(1)  rst=on  en=on  dbl_ovrd=off  block_type=register
  Register1 : xbsIndex_r4/Register  init=init(2)  rst=on  en=on  dbl_ovrd=off  block_type=register
  Register2 : xbsIndex_r4/Register  init=init(3)  rst=on  en=on  dbl_ovrd=off  block_type=register
  Register3 : xbsIndex_r4/Register  init=init(4)  rst=on  en=on  dbl_ovrd=off  block_type=register
  Register4 : xbsIndex_r4/Register  init=init(5)  rst=on  en=on  dbl_ovrd=off  block_type=register
  Register5 : xbsIndex_r4/Register  init=init(6)  rst=on  en=on  dbl_ovrd=off  block_type=register
  Register6 : xbsIndex_r4/Register  init=init(7)  rst=on  en=on  dbl_ovrd=off  block_type=register
  Register7 : xbsIndex_r4/Register  init=init(8)  rst=on  en=on  dbl_ovrd=off  block_type=register
  data_out : Outport
  wires:
  Register/1 -> Register1/1
  enable_in/1 -> Register7/3, Register6/3, Register5/3, Register4/3, Register3/3, Register2/3, Register1/3, Register/3
  Register7/1 -> data_out/1
  Register1/1 -> Register2/1
  Register2/1 -> Register3/1
  Register3/1 -> Register4/1
  Register5/1 -> Register6/1
  Register6/1 -> Register7/1
  Register4/1 -> Register5/1
  reset_in/1 -> Register/2, Register1/2, Register2/2, Register3/2, Register4/2, Register7/2, Register6/2, Register5/2
  data_in/1 -> Register/1

== system sim_model/channelizer/poly_phase_filter1/filter_pipeline_89_taps3/8_taps7/one_tab_8/ring_buffer_8 ==
  reset_in : Inport
  enable_in : Inport  Port=2
  data_in : Inport  Port=3
  Register : xbsIndex_r4/Register  init=init(1)  rst=on  en=on  dbl_ovrd=off  block_type=register
  Register1 : xbsIndex_r4/Register  init=init(2)  rst=on  en=on  dbl_ovrd=off  block_type=register
  Register2 : xbsIndex_r4/Register  init=init(3)  rst=on  en=on  dbl_ovrd=off  block_type=register
  Register3 : xbsIndex_r4/Register  init=init(4)  rst=on  en=on  dbl_ovrd=off  block_type=register
  Register4 : xbsIndex_r4/Register  init=init(5)  rst=on  en=on  dbl_ovrd=off  block_type=register
  Register5 : xbsIndex_r4/Register  init=init(6)  rst=on  en=on  dbl_ovrd=off  block_type=register
  Register6 : xbsIndex_r4/Register  init=init(7)  rst=on  en=on  dbl_ovrd=off  block_type=register
  Register7 : xbsIndex_r4/Register  init=init(8)  rst=on  en=on  dbl_ovrd=off  block_type=register
  data_out : Outport
  wires:
  Register/1 -> Register1/1
  enable_in/1 -> Register7/3, Register6/3, Register5/3, Register4/3, Register3/3, Register2/3, Register1/3, Register/3
  Register7/1 -> data_out/1
  Register1/1 -> Register2/1
  Register2/1 -> Register3/1
  Register3/1 -> Register4/1
  Register5/1 -> Register6/1
  Register6/1 -> Register7/1
  Register4/1 -> Register5/1
  reset_in/1 -> Register/2, Register1/2, Register2/2, Register3/2, Register4/2, Register7/2, Register6/2, Register5/2
  data_in/1 -> Register/1
